simulink model "system_approach_final_with_SVM"  (R2019a)
settings: Solver=ode23tb  StartTime=0.0  StopTime=18  RelTol=1e-6  AbsTol=1e-6
InitFcn:
  | Tpwm=1/10000;
undefined symbols (not defined in the file): dEgdT, EgRef, gcbh, k1, Rsh_array5pc, sigbuilder_block, sps_rtmsupport, Tref_K, VT_ref
libraries: powerlib x16, spsPVarrayModel x3, powerlib_meascontrol x2, simulink x2
(part 5 of 5)

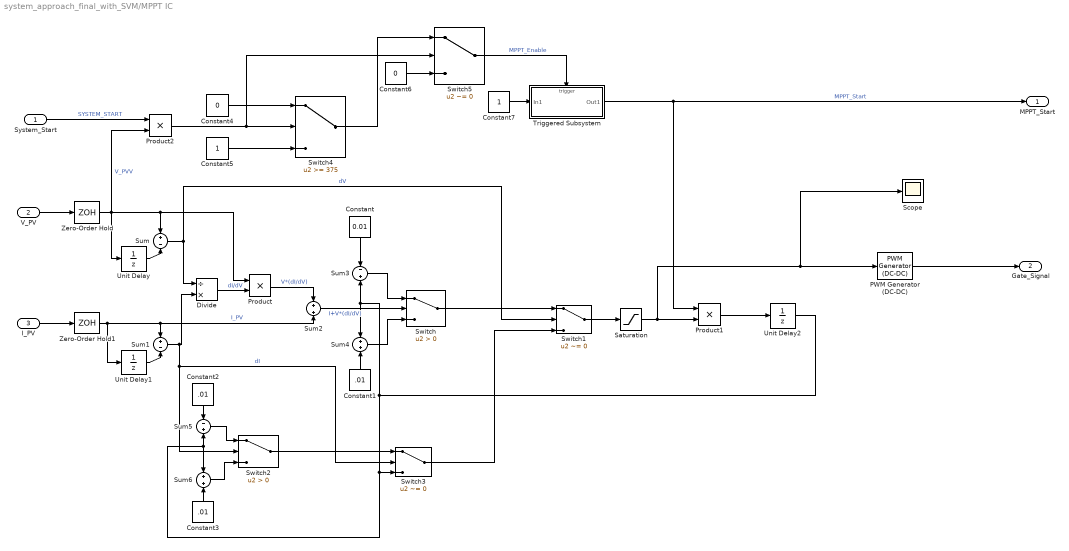
== system system_approach_final_with_SVM/MPPT IC ==
  System_Start : Inport
  V_PV : Inport  Port=2
  I_PV : Inport  Port=3
  Constant : Constant  Value=0.01
  Constant1 : Constant  Value=.01
  Constant2 : Constant  Value=.01
  Constant3 : Constant  Value=.01
  Constant4 : Constant  Value=0
  Constant5 : Constant
  Constant6 : Constant  Value=0
  Constant7 : Constant
  Divide : Product  Inputs=/*
  PWM Generator (DC-DC) : powerlib_meascontrol/Pulse & Signal Generators/PWM Generator (DC-DC)  Fsw=10000  Ts=0
      settings: SourceProductName=Simscape Electrical
  Product : Product
  Product1 : Product
  Product2 : Product
  Saturation : Saturate  UpperLimit=.95  LowerLimit=.01
  Scope : Scope
  Sum : Sum  Inputs=+-
  Sum1 : Sum  Inputs=+-
  Sum2 : Sum
  Sum3 : Sum  Inputs=-+
  Sum4 : Sum
  Sum5 : Sum  Inputs=-+
  Sum6 : Sum
  Switch : Switch  Criteria=u2 > Threshold
  Switch1 : Switch  Criteria=u2 ~= 0
  Switch2 : Switch  Criteria=u2 > Threshold
  Switch3 : Switch  Criteria=u2 ~= 0
  Switch4 : Switch  Threshold=375
  Switch5 : Switch  Criteria=u2 ~= 0  Threshold=375
  Triggered Subsystem : Subsystem  TreatAsAtomicUnit=on
  Unit Delay : UnitDelay  SampleTime=-1  HasFrameUpgradeWarning=on
  Unit Delay1 : UnitDelay  SampleTime=-1  HasFrameUpgradeWarning=on
  Unit Delay2 : UnitDelay  SampleTime=-1  HasFrameUpgradeWarning=on
  Zero-Order Hold : ZeroOrderHold  SampleTime=Tpwm
  Zero-Order Hold1 : ZeroOrderHold  SampleTime=Tpwm
  MPPT_Start : Outport
  Gate_Signal : Outport  Port=2
  wires:
  V_PV/1 -> Zero-Order Hold/1
  I_PV/1 -> Zero-Order Hold1/1
  Zero-Order Hold/1 -> Unit Delay/1, Product2/2, Sum/1, Product/1  "V_PVV"
  Unit Delay/1 -> Sum/2
  Sum/1 -> Switch1/2, Divide/1  "dV"
  Zero-Order Hold1/1 -> Sum1/1, Sum2/2, Unit Delay1/1  "I_PV"
  Unit Delay1/1 -> Sum1/2
  Sum1/1 -> Switch3/2, Switch2/2, Divide/2  "dI"
  Divide/1 -> Product/2  "dI/dV"
  Product/1 -> Sum2/1  "V*(dI/dV)"
  Sum2/1 -> Switch/2  "I+V*(dI/dV)"
  Constant/1 -> Sum3/1
  Sum3/1 -> Switch/1
  Constant1/1 -> Sum4/2
  Sum4/1 -> Switch/3
  Switch/1 -> Switch1/1
  Sum5/1 -> Switch2/1
  Constant2/1 -> Sum5/1
  Sum6/1 -> Switch2/3
  Constant3/1 -> Sum6/2
  Switch2/1 -> Switch3/1
  Switch3/1 -> Switch1/3
  Switch1/1 -> Saturation/1
  Saturation/1 -> Scope/1, PWM Generator (DC-DC)/1, Product1/2
  Unit Delay2/1 -> Sum4/1, Sum3/2, Switch3/3, Sum6/1, Sum5/2
  System_Start/1 -> Product2/1  "SYSTEM_START"
  Product2/1 -> Switch5/2, Switch4/2
  Constant4/1 -> Switch4/1
  Constant5/1 -> Switch4/3
  Switch4/1 -> Switch5/1
  Constant6/1 -> Switch5/3
  Switch5/1 -> Triggered Subsystem/Trigger  "MPPT_Enable"
  Constant7/1 -> Triggered Subsystem/1(In1)
  Triggered Subsystem/1(Out1) -> Product1/1, MPPT_Start/1  "MPPT_Start"
  PWM Generator (DC-DC)/1 -> Gate_Signal/1
  Product1/1 -> Unit Delay2/1

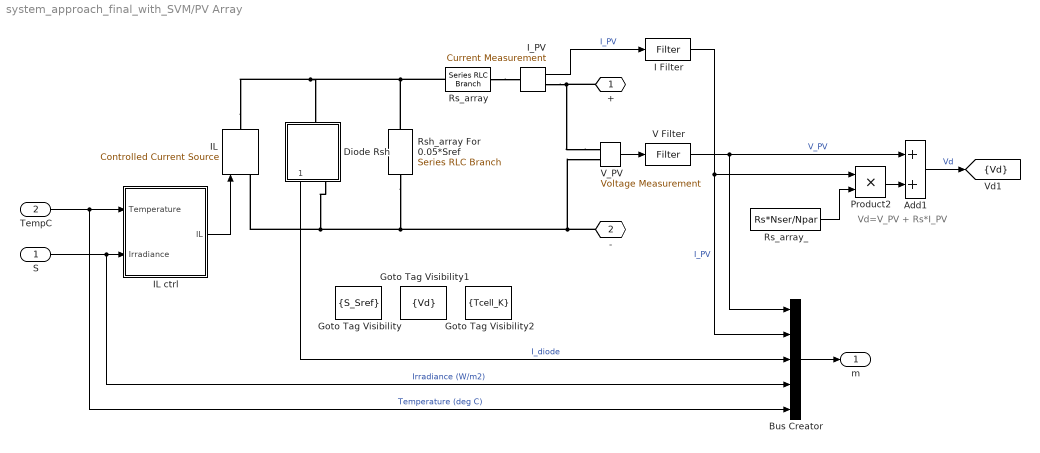
== system system_approach_final_with_SVM/PV Array ==
  note: Vd=V_PV + Rs*I_PV
  S : Inport
  TempC : Inport  Port=2
  Add1 : Sum
  Bus Creator : BusCreator  Inputs=5
  Diode Rsh : Subsystem
      mask Display:
      | plot(-75,-50,100,150, [-15 -15 43 -15 -15 -75],[50 8 50 92 50 50], ...
      |     [43 43],[8 94],[100 43], [50 50])
  Goto Tag Visibility : GotoTagVisibility  GotoTag=S_Sref
  Goto Tag Visibility1 : GotoTagVisibility  GotoTag=Vd
  Goto Tag Visibility2 : GotoTagVisibility  GotoTag=Tcell_K
  I Filter : spsPVarrayModel/Filter  SystemSampleTime=-1  VariantControl=Variant1
      settings: SourceProductName=Simscape Electrical  SourceProductBaseCode=PS
  IL : powerlib/Electrical Sources/Controlled Current Source  Initialize=on  Source_Type=AC  Amplitude=0  Phase=0  Frequency=0  Measurements=None
      settings: SourceProductName=Simscape Electrical
  IL ctrl : Subsystem
  I_PV : powerlib/Measurements/Current Measurement  PhasorSimulation=off  OutputType=Complex  PSBequivalent=0
      settings: SourceProductName=Simscape Electrical
  Product2 : Product  Inputs=**  RndMeth=Zero
  Rs_array : powerlib/Elements/Series RLC Branch  LConnTagsString=__new0  RConnTagsString=__new0  BranchType=R  Resistance=Rs*Nser/Npar  Inductance=1e-3  SetiL0=off  InitialCurrent=0  Capacitance=1e-6  Setx0=off  InitialVoltage=0  Measurements=None
      settings: SourceProductName=Simscape Electrical
  Rs_array_ : Constant  Value=Rs*Nser/Npar
  Rsh_array For 0.05*Sref : powerlib/Elements/Series RLC Branch  LConnTagsString=__new0  RConnTagsString=__new0  BranchType=R  Resistance=Rsh_array5pc  Inductance=1e-3  SetiL0=off  InitialCurrent=0  Capacitance=1e-6  Setx0=off  InitialVoltage=0  Measurements=None
      settings: SourceProductName=Simscape Electrical
  V Filter : spsPVarrayModel/Filter  SystemSampleTime=-1  VariantControl=Variant1
      settings: SourceProductName=Simscape Electrical  SourceProductBaseCode=PS
  V_PV : powerlib/Measurements/Voltage Measurement  PhasorSimulation=off  OutputType=Complex  PSBequivalent=0
      settings: SourceProductName=Simscape Electrical
  + : PMIOPort  Side=Right
  - : PMIOPort  Port=2  Side=Right
  m : Outport
  tag scope: Vd=scoped
  wires:
  V Filter/1 -> Add1/1, Bus Creator/1  "V_PV"
  I Filter/1 -> Product2/1, Bus Creator/2  "I_PV"
  V_PV/1 -> V Filter/1
  IL ctrl/1(IL) -> IL/1
  Bus Creator/1 -> m/1
  Rs_array_/1 -> Product2/2
  Product2/1 -> Add1/2
  I_PV/1 -> I Filter/1  "I_PV"
  Add1/1 -> [Vd]  "Vd"
  Diode Rsh/1(Idiode) -> Bus Creator/3  "I_diode"
  S/1 -> Bus Creator/4, IL ctrl/2(Irradiance)  "Irradiance (W/m2)"
  TempC/1 -> IL ctrl/1(Temperature), Bus Creator/5  "Temperature (deg C)"
  connections:
  Rs_array/RConn1 -- I_PV/LConn1
  IL/LConn1 -- Diode Rsh/RConn1 -- Rsh_array For 0.05*Sref/RConn1 -- -/RConn1 -- V_PV/LConn2
  IL/RConn1 -- Rsh_array For 0.05*Sref/LConn1 -- Rs_array/LConn1 -- Diode Rsh/LConn1
  V_PV/LConn1 -- I_PV/RConn1 -- +/RConn1

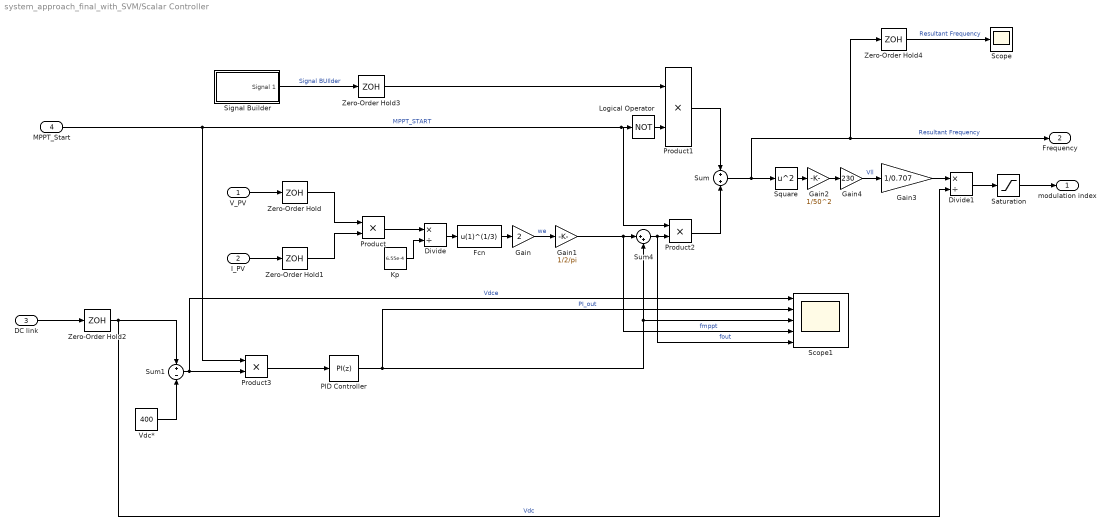
== system system_approach_final_with_SVM/Scalar Controller ==
  V_PV : Inport
  I_PV : Inport  Port=2
  DC link : Inport  Port=3
  MPPT_Start : Inport  Port=4
  Divide : Product  Inputs=*/
  Divide1 : Product  Inputs=*/
  Fcn : Fcn  Expr=u(1)^(1/3)
  Gain : Gain  Gain=2
  Gain1 : Gain  Gain=1/2/pi
  Gain2 : Gain  Gain=1/50^2
  Gain3 : Gain  Gain=1/0.707
  Gain4 : Gain  Gain=230
  Kp : Constant  Value=6.55e-4
  Logical Operator : Logic  Operator=NOT  AllPortsSameDT=off  OutDataTypeStr=boolean
  PID Controller : simulink/Continuous/PID Controller  Controller=PI  Form=Parallel  TimeDomain=Discrete-time  SampleTime=-1  IntegratorMethod=Forward Euler  FilterMethod=Forward Euler  ControllerParametersSource=internal  P=.1  I=3  D=0  UseFilter=on  N=100  TunerSelectOption=Transfer Function Based (PID Tuner App)  InitialConditionSource=internal  InitialConditionForIntegrator=0  InitialConditionForFilter=0  DifferentiatorICPrevScaledInput=0  ExternalReset=none  TrackingMode=off  Kt=1  LimitOutput=off  UpperSaturationLimit=inf  LowerSaturationLimit=-inf  LinearizeAsGain=on  AntiWindupMode=none  Kb=1  POutMin=[]  POutMax=[]  IOutMin=[]  IOutMax=[]  DOutMin=[]  DOutMax=[]  NOutMin=[]  NOutMax=[]  SumOutMin=[]  SumOutMax=[]  SaturationOutMin=[]  SaturationOutMax=[]  PParamMin=[]  PParamMax=[]  IParamMin=[]  IParamMax=[]  DParamMin=[]  DParamMax=[]  NParamMin=[]  NParamMax=[]  KbParamMin=[]  KbParamMax=[]  KtParamMin=[]  KtParamMax=[]  KbOutMin=[]  KbOutMax=[]  KtOutMin=[]  KtOutMax=[]  IntegratorOutMin=[]  IntegratorOutMax=[]  FilterOutMin=[]  FilterOutMax=[]  SumI1OutMin=[]  SumI1OutMax=[]  SumI2OutMin=[]  SumI2OutMax=[]  SumI3OutMin=[]  SumI3OutMax=[]  SumI4OutMin=[]  SumI4OutMax=[]  SumDOutMin=[]  SumDOutMax=[]  DifferentiatorOutMin=[]  DifferentiatorOutMax=[]  FilterDiffOutCoefMin=[]  FilterDiffOutCoefMax=[]  ReciprocalOutMin=[]  ReciprocalOutMax=[]  SumDenOutMin=[]  SumDenOutMax=[]  SumNumOutMin=[]  SumNumOutMax=[]  DivideOutMin=[]  DivideOutMax=[]  IntegratorContinuousStateAttributes=''  IntegratorStateMustResolveToSignalObject=off  IntegratorRTWStateStorageClass=Auto  FilterContinuousStateAttributes=''  FilterStateMustResolveToSignalObject=off  FilterRTWStateStorageClass=Auto  ParallelPVariant=InternalParameters  IdealPVariant=Disabled  IVariant=InternalParameters  DVariant=Disabled  IntegratorVariant=Discrete  SatVariant=Disabled  AWVariant=Passthrough  PCopyVariant=Disabled  TRVariant=Disabled  FdbkBlocksVariant=Forward  IdealPFdbkVariant=Disabled  SatFdbkVariant=Disabled  DerivativeFilterVariant=Disabled  NVariant=Disabled  NCopyVariant=Disabled_SignalSpec  FilterICVariant=Disabled  IntegratorICVariant=InternalICs  ExternalResetVariant=Disabled  TRSumVariant=Passthrough  SumFdbkVariant=Disabled  SumVariant=Sum_PI
  Product{,1..3} (4 alike) : Product
  Saturation : Saturate  UpperLimit=1  LowerLimit=0
  Scope : Scope
  Scope1 : Scope  NumInputPorts=5
  Signal Builder : Subsystem  Tag=STV Subsys  LoadFcn=sigbuilder_block('load',[5.5 30 949 418 ]);  StartFcn=sigbuilder_block('start');  StopFcn=sigbuilder_block('stop');  ClipboardFcn=sigbuilder_block('clipboard');  mask(Sigbuilder block){tuvar=[0:10]}
      mask help: Simulink:masks:SigbuilderBlock_MD
      mask init:
      | if ~strcmp(get_param(bdroot(gcbh),'SimulationStatus'),'stopped') tuvar = sigbuilder_block('maskInit'); end
      settings: CopyFcn=sigbuilder_block('copy');  DeleteFcn=sigbuilder_block('delete');  ModelCloseFcn=sigbuilder_block('modelClose');  PreSaveFcn=sigbuilder_block('preSave');  PauseFcn=sigbuilder_block('pause');  ContinueFcn=sigbuilder_block('continue');  NameChangeFcn=sigbuilder_block('namechange');  OpenFcn=sigbuilder_block('open',[0 30 960 455.5 ]);  CloseFcn=sigbuilder_block('close');
      mask Display: plot(0, 0, 100, 100,[2, 2, 32, 32, 2], [68, 8, 8, 68, 68],[32, 2], [38, 38], [32, 19, 2],[53, 60, 44], [32, 17, 17, 2],[16, 16, 31, 31]);txt = getActiveGroup(gcbh);text(2, 100, txt,'verticalAlignment', 'top');
  Square : Math  Operator=square  SaturateOnIntegerOverflow=on
  Sum : Sum
  Sum1 : Sum  Inputs=+-
  Sum4 : Sum  Inputs=|++
  Vdc* : Constant  Value=400
  Zero-Order Hold{,1..3} (4 alike) : ZeroOrderHold  SampleTime=4*Tpwm
  Zero-Order Hold4 : ZeroOrderHold  SampleTime=Tpwm
  modulation index : Outport
  Frequency : Outport  Port=2
  wires:
  I_PV/1 -> Zero-Order Hold1/1
  V_PV/1 -> Zero-Order Hold/1
  Zero-Order Hold/1 -> Product/1
  Zero-Order Hold1/1 -> Product/2
  Product/1 -> Divide/1
  Kp/1 -> Divide/2
  Divide/1 -> Fcn/1
  Fcn/1 -> Gain/1
  Gain/1 -> Gain1/1  "we"
  Gain1/1 -> Scope1/4, Sum4/1  "fmppt"
  DC link/1 -> Zero-Order Hold2/1
  Gain4/1 -> Gain3/1  "Vll"
  Gain3/1 -> Divide1/1
  Zero-Order Hold2/1 -> Sum1/1, Divide1/2  "Vdc"
  Divide1/1 -> Saturation/1
  Saturation/1 -> modulation index/1
  MPPT_Start/1 -> Product3/1, Logical Operator/1, Product2/1  "MPPT_START"
  Signal Builder/1(Signal 1) -> Zero-Order Hold3/1  "Signal BUIlder"
  Logical Operator/1 -> Product1/2
  Product1/1 -> Sum/1
  Product2/1 -> Sum/2
  Sum/1 -> Square/1, Zero-Order Hold4/1, Frequency/1  "Resultant Frequency"
  Zero-Order Hold3/1 -> Product1/1
  Vdc*/1 -> Sum1/2
  Sum4/1 -> Scope1/5, Product2/2  "fout"
  Sum1/1 -> Scope1/1, Product3/2  "Vdce"
  Product3/1 -> PID Controller/1
  PID Controller/1 -> Sum4/2, Scope1/3, Scope1/2  "PI_out"
  Zero-Order Hold4/1 -> Scope/1  "Resultant Frequency"
  Square/1 -> Gain2/1
  Gain2/1 -> Gain4/1

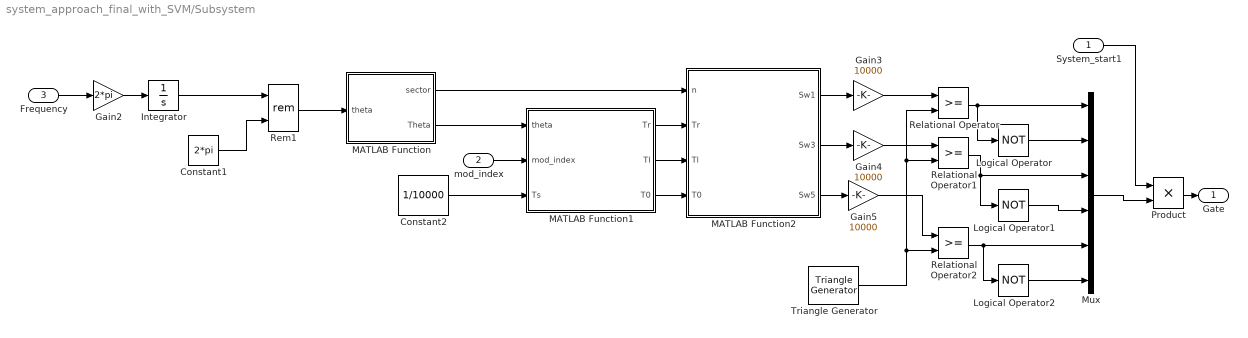
== system system_approach_final_with_SVM/Subsystem ==
  System_start1 : Inport
  mod_index : Inport  Port=2
  "Frequency " : Inport  Port=3
  Constant1 : Constant  Value=2*pi
  Constant2 : Constant  Value=1/10000
  Gain2 : Gain  Gain=2*pi
  Gain3 : Gain  Gain=10000
  Gain4 : Gain  Gain=10000
  Gain5 : Gain  Gain=10000
  Integrator : Integrator
  Logical Operator : Logic  Operator=NOT  AllPortsSameDT=off  OutDataTypeStr=boolean
  Logical Operator1 : Logic  Operator=NOT  AllPortsSameDT=off  OutDataTypeStr=boolean
  Logical Operator2 : Logic  Operator=NOT  AllPortsSameDT=off  OutDataTypeStr=boolean
  MATLAB Function : MATLAB Function  TreatAsAtomicUnit=on
  MATLAB Function1 : MATLAB Function  TreatAsAtomicUnit=on
  MATLAB Function2 : MATLAB Function  TreatAsAtomicUnit=on
  Mux : Mux  Inputs=6
  Product : Product
  Relational Operator : RelationalOperator  OutDataTypeStr=boolean  RndMeth=Simplest
  Relational Operator1 : RelationalOperator  OutDataTypeStr=boolean  RndMeth=Simplest
  Relational Operator2 : RelationalOperator  OutDataTypeStr=boolean  RndMeth=Simplest
  Rem1 : Math  Operator=rem  SaturateOnIntegerOverflow=on
  Triangle Generator : powerlib_meascontrol/Pulse & Signal Generators/Triangle Generator  Freq=10000  Phase=0  Ts=0
      settings: SourceProductName=Simscape Electrical
  Gate : Outport
  wires:
  "Frequency "/1 -> Gain2/1
  MATLAB Function2/1(Sw1) -> Gain3/1
  MATLAB Function/2(Theta) -> MATLAB Function1/1(theta)
  Gain5/1 -> Relational Operator2/1
  Rem1/1 -> MATLAB Function/1(theta)
  MATLAB Function1/1(Tr) -> MATLAB Function2/2(Tr)
  Relational Operator1/1 -> Logical Operator1/1, Mux/3
  Gain3/1 -> Relational Operator/1
  MATLAB Function/1(sector) -> MATLAB Function2/1(n)
  Gain2/1 -> Integrator/1
  Constant1/1 -> Rem1/2
  Relational Operator/1 -> Logical Operator/1, Mux/1
  Integrator/1 -> Rem1/1
  Constant2/1 -> MATLAB Function1/3(Ts)
  Triangle Generator/1 -> Relational Operator/2, Relational Operator1/2, Relational Operator2/2
  Gain4/1 -> Relational Operator1/1
  Logical Operator1/1 -> Mux/4
  MATLAB Function2/2(Sw3) -> Gain4/1
  MATLAB Function1/2(Tl) -> MATLAB Function2/3(Tl)
  MATLAB Function1/3(T0) -> MATLAB Function2/4(T0)
  MATLAB Function2/3(Sw5) -> Gain5/1
  Relational Operator2/1 -> Mux/5, Logical Operator2/1
  Logical Operator/1 -> Mux/2
  Logical Operator2/1 -> Mux/6
  mod_index/1 -> MATLAB Function1/2(mod_index)
  Product/1 -> Gate/1
  Mux/1 -> Product/2
  System_start1/1 -> Product/1

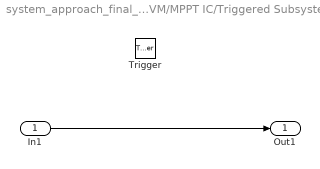
== system system_approach_final_with_SVM/MPPT IC/Triggered Subsystem ==
  In1 : Inport
  Trigger : TriggerPort  VariantControl=Variant
  Out1 : Outport
  wires:
  In1/1 -> Out1/1

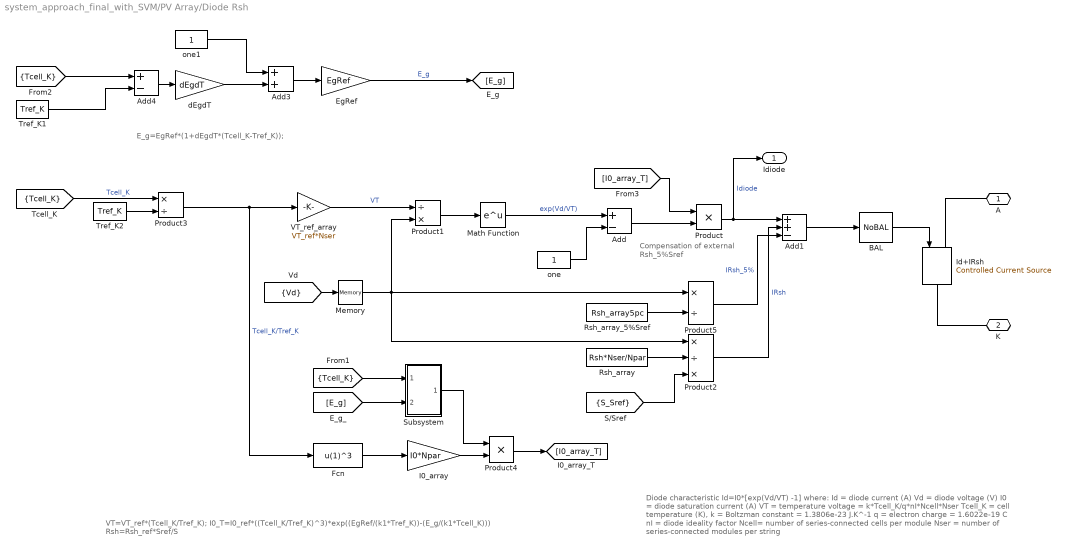
== system system_approach_final_with_SVM/PV Array/Diode Rsh ==
  note: Compensation of
      | external Rsh_5%Sref
  note: Diode characteristic
      |    Id=I0*[exp(Vd/VT) -1]
      |
      | where:
      |      Id = diode current (A)
      |      Vd = diode voltage (V)
      |      I0 = diode saturation current (A)
      |      VT = temperature voltage = k*Tcell_K/q*nI*Ncell*Nser
      | Tcell_K = cell temperature (K),
      |       k = Boltzman constant = 1.3806e-23 J.K^-1
      |       q = electron charge = 1.6022e-19 C
      |      nI = diode ideality factor
      |    Ncell= number of series-connected cells per module
      |    Nser = number of series-connected modules per string
  note: VT=VT_ref*(Tcell_K/Tref_K);
      | I0_T=I0_ref*((Tcell_K/Tref_K)^3)*exp((EgRef/(k1*Tref_K))-(E_g/(k1*Tcell_K)))
      | Rsh=Rsh_ref*Sref/S
  note: E_g=EgRef*(1+dEgdT*(Tcell_K-Tref_K));
  Add : Sum  Inputs=+-
  Add1 : Sum  Inputs=++-
  Add3 : Sum
  Add4 : Sum  Inputs=+-
  BAL : spsPVarrayModel/NoBAL  SystemSampleTime=-1  VariantControl=NoBAL
      settings: SourceProductName=Simscape Electrical  SourceProductBaseCode=PS
  EgRef : Gain  Gain=EgRef
  Fcn : Fcn  Expr=u(1)^3
  I0_array : Gain  Gain=I0*Npar
  Id+IRsh : powerlib/Electrical Sources/Controlled Current Source  Initialize=on  Source_Type=AC  Amplitude=0  Phase=0  Frequency=0  Measurements=None
      settings: SourceProductName=Simscape Electrical
  Math Function : Math  SaturateOnIntegerOverflow=on
  Memory : Memory  InheritSampleTime=on
  Product : Product  RndMeth=Zero
  Product1 : Product  Inputs=/*  RndMeth=Zero
  Product2 : Product  Inputs=*/*  RndMeth=Zero
  Product3 : Product  Inputs=*/  RndMeth=Zero
  Product4 : Product  Inputs=**  RndMeth=Zero
  Product5 : Product  Inputs=*/  RndMeth=Zero
  Rsh_array : Constant  Value=Rsh*Nser/Npar
  Rsh_array_5%Sref : Constant  Value=Rsh_array5pc
  Subsystem : Subsystem
  Tref_K1 : Constant  Value=Tref_K
  Tref_K2 : Constant  Value=Tref_K
  VT_ref_array : Gain  Gain=VT_ref*Nser
  dEgdT : Gain  Gain=dEgdT
  one : Constant
  one1 : Constant
  A : PMIOPort  Side=Left
  K : PMIOPort  Port=2  Side=Right
  Idiode : Outport
  wires:
  BAL/1 -> Id+IRsh/1
  Add1/1 -> BAL/1
  Product5/1 -> Add1/3  "IRsh_5%"
  Rsh_array_5%Sref/1 -> Product5/2
  Math Function/1 -> Add/1  "exp(Vd/VT)"
  Product2/1 -> Add1/2  "IRsh"
  Product/1 -> Add1/1, Idiode/1  "Idiode"
  Product1/1 -> Math Function/1
  one/1 -> Add/2
  Rsh_array/1 -> Product2/2
  [Tcell_K] -> Product3/1  "Tcell_K"
  Product3/1 -> VT_ref_array/1, Fcn/1  "Tcell_K/Tref_K"
  one1/1 -> Add3/1
  Add4/1 -> dEgdT/1
  dEgdT/1 -> Add3/2
  Add3/1 -> EgRef/1
  EgRef/1 -> [E_g]  "E_g"
  I0_array/1 -> Product4/2
  Fcn/1 -> I0_array/1
  [Tcell_K] -> Add4/1
  Tref_K1/1 -> Add4/2
  Subsystem/1(exp) -> Product4/1
  [Tcell_K] -> Subsystem/1(Tcell_K)
  [E_g] -> Subsystem/2(E_g)
  Tref_K2/1 -> Product3/2
  Product4/1 -> [I0_array_T]
  Add/1 -> Product/2
  VT_ref_array/1 -> Product1/1  "VT"
  [I0_array_T] -> Product/1
  [S_Sref] -> Product2/3
  [Vd] -> Memory/1
  Memory/1 -> Product5/1, Product2/1, Product1/2
  connections:
  Id+IRsh/RConn1 -- K/RConn1
  A/RConn1 -- Id+IRsh/LConn1

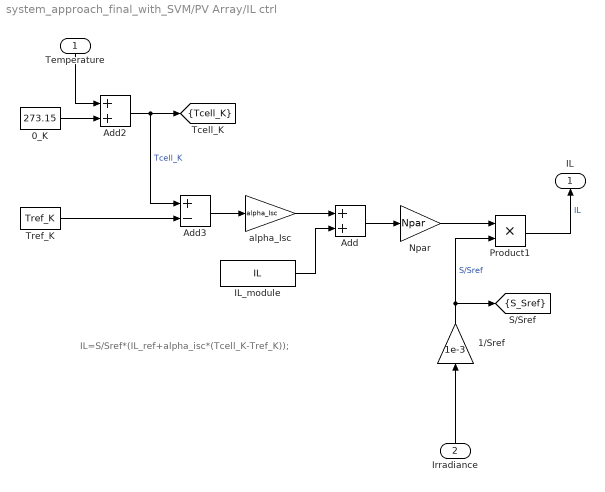
== system system_approach_final_with_SVM/PV Array/IL ctrl ==
  note: IL=S/Sref*(IL_ref+alpha_isc*(Tcell_K-Tref_K));
  Temperature : Inport
  Irradiance : Inport  Port=2
  0_K : Constant  Value=273.15
  1/Sref : Gain  Gain=1e-3
  Add : Sum
  Add2 : Sum
  Add3 : Sum  Inputs=+-
  IL_module : Constant  Value=IL
  Npar : Gain  Gain=Npar
  Product1 : Product  Inputs=**  RndMeth=Zero
  Tref_K : Constant  Value=Tref_K
  alpha_Isc : Gain  Gain=alpha_Isc
  IL : Outport
  tag scope: S_Sref=scoped, Tcell_K=scoped
  wires:
  Temperature/1 -> Add2/1
  Irradiance/1 -> 1/Sref/1
  alpha_Isc/1 -> Add/1
  Add3/1 -> alpha_Isc/1
  Tref_K/1 -> Add3/2
  Product1/1 -> IL/1  "IL"
  IL_module/1 -> Add/2
  0_K/1 -> Add2/2
  Add/1 -> Npar/1
  Add2/1 -> Add3/1, [Tcell_K]  "Tcell_K"
  Npar/1 -> Product1/1
  1/Sref/1 -> Product1/2, [S_Sref]  "S/Sref"

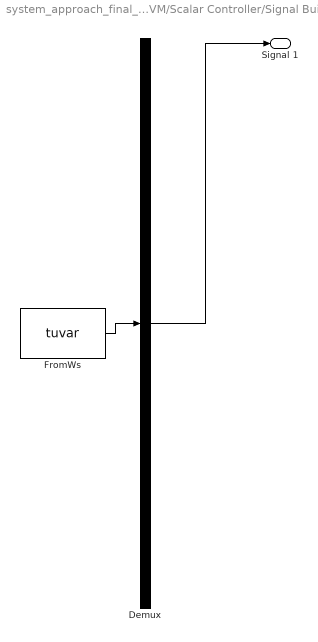
== system system_approach_final_with_SVM/Scalar Controller/Signal Builder ==
  Demux : Demux  Tag=STV Demux  Outputs=1
  FromWs : FromWorkspace  Tag=STV FromWs  VariableName=tuvar  SampleTime=0
      SigBuilderData=|
      | common.afterFinalStr = 'Extrapolate'
      | common.sampleTime = 0
      | dataSet.timeRange = [0 10]
      | dataSet.name = 'Group 1'
      | sbobj.Groups.Name = 'Group 1'
      | sbobj.Groups.Signals.Name = 'Signal 1'
      | sbobj.Groups.Signals.XData = [0 0.5 2 10]
      | sbobj.Groups.Signals.YData = [0 0 50 50]
  Signal 1 : Outport  Tag=STV Outport
  wires:
  Demux/1 -> Signal 1/1
  FromWs/1 -> Demux/1

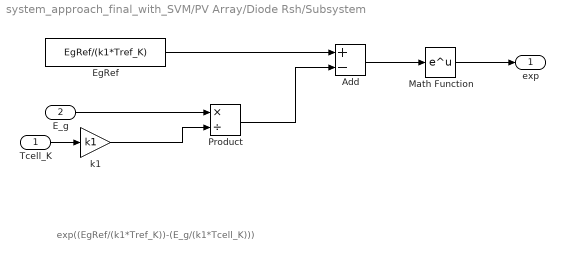
== system system_approach_final_with_SVM/PV Array/Diode Rsh/Subsystem ==
  note: exp((EgRef/(k1*Tref_K))-(E_g/(k1*Tcell_K)))
  Tcell_K : Inport
  E_g : Inport  Port=2
  Add : Sum  Inputs=+-
  EgRef : Constant  Value=EgRef/(k1*Tref_K)
  Math Function : Math  SaturateOnIntegerOverflow=on
  Product : Product  Inputs=*/
  k1 : Gain  Gain=k1
  exp : Outport
  wires:
  EgRef/1 -> Add/1
  E_g/1 -> Product/1
  Tcell_K/1 -> k1/1
  k1/1 -> Product/2
  Product/1 -> Add/2
  Add/1 -> Math Function/1
  Math Function/1 -> exp/1

== matlab function system_approach_final_with_SVM/Subsystem/MATLAB Function ==
  data: theta input; sector output; Theta output
function [sector,Theta]= fcn(theta)
sector=0;
Theta=0;
if(theta>=0 && theta<pi/3)
    sector=1;
    Theta=theta;
end
if(theta>=pi/3 && theta<2*pi/3)
    sector=2;
    Theta=theta-pi/3;
end

if(theta>=2*pi/3 && theta<pi)
    sector=3;
    Theta=theta-2*pi/3;
end

if(theta>=3*pi/3 && theta<4*pi/3)
    sector=4;
    Theta=theta-3*pi/3;
end
if(theta>=4*pi/3 && theta<5*pi/3)
    sector=5;
    Theta=theta-4*pi/3;
end

if(theta>=5*pi/3 && theta<2*pi)
    sector=6;
    Theta=theta-5*pi/3;
end

== matlab function system_approach_final_with_SVM/Subsystem/MATLAB Function1 ==
  data: theta input; Tr output; mod_index input; Ts input; Tl output; T0 output
function [Tr,Tl,T0]= switch_time_calculation(theta,mod_index,Ts)
Tr=mod_index*Ts*sin(pi/3-theta);
Tl=mod_index*Ts*sin(theta);
T0=Ts-Tr-Tl;

== matlab function system_approach_final_with_SVM/Subsystem/MATLAB Function2 ==
  data: n input; Tr input; Tl input; Sw1 output; T0 input; Sw3 output; Sw5 output
function [Sw1,Sw3,Sw5]= Time_for_each_leg(n,Tr,Tl,T0)

%#codegen
Sw1=0;
Sw3=0;
Sw5=0;
if (n==1)
Sw1=Tl+Tr+T0/2;
Sw3=Tl+T0/2;
Sw5=T0/2;
end
if (n==2)
Sw1=Tr+T0/2;
Sw3=Tl+Tr+T0/2;
Sw5=T0/2;
end
if (n==3)
Sw1=T0/2;
Sw3=Tr+Tl+T0/2;
Sw5=Tl+T0/2;
end
if (n==4)
Sw1=T0/2;
Sw3=Tr+T0/2;
Sw5=Tr+Tl+T0/2;
end
if (n==5)
Sw1=Tl+T0/2;
Sw3=T0/2;
Sw5=Tr+Tl+T0/2;
end
if (n==6)
Sw1=Tl+Tr+T0/2;
Sw3=T0/2;
Sw5=Tr+T0/2;
end
